simulink model "main"  (R2022b)
settings: Solver=VariableStepAuto  StartTime=0.0  StopTime=10.0  RelTol=1e-3
model workspace (MAT data in the model file):
  a0 = 1
  a1 = 1
  a2 = 1
settings Model: Creator=markm  LastModifiedBy=markm

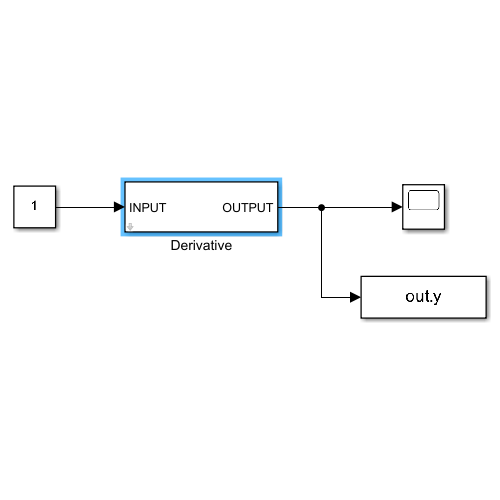
[thumbnail: Simulink's stored preview of the top-level diagram]
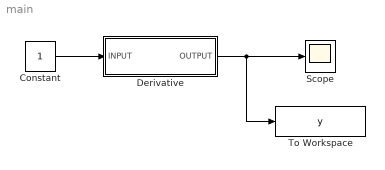
== system main ==
  Constant : Constant
  Derivative : Subsystem  mask{a2=1, a1=2, a0=3}
  Scope : Scope
  To Workspace : ToWorkspace  VariableName=y  SaveFormat=Timeseries  SampleTime=-1
  wires:
  Derivative/1(OUTPUT) -> To Workspace/1, Scope/1
  Constant/1 -> Derivative/1(INPUT)

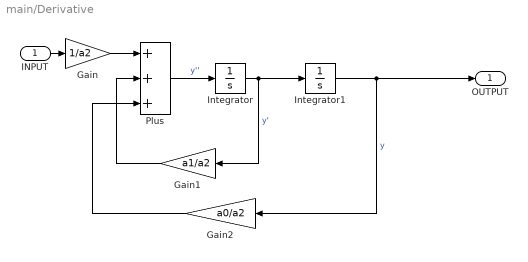
== system main/Derivative ==
  INPUT : Inport
  Gain : Gain  Gain=1/a2
  Gain1 : Gain  Gain=a1/a2
  Gain2 : Gain  Gain=a0/a2
  Integrator : Integrator
  Integrator1 : Integrator
  Plus : Sum  Inputs=+++
  OUTPUT : Outport
  wires:
  Gain1/1 -> Plus/2
  Integrator/1 -> Gain1/1, Integrator1/1  "y'"
  Integrator1/1 -> OUTPUT/1, Gain2/1  "y"
  Gain2/1 -> Plus/3
  Plus/1 -> Integrator/1  "y''"
  INPUT/1 -> Gain/1
  Gain/1 -> Plus/1
